simulink library "FMLibrary_v2"  (R2016b)
settings: Solver=ode45  StartTime=0.0  StopTime=10.0  RelTol=1e-3
undefined symbols (not defined in the file or in its folder): ActuatorStruct, drivePeakCurrent, IdxJoint, JointPositionGuardMax_rad, JointPositionGuardMin_rad, Lb, Lf, Lu, motorTorqueConstant, RobotStruct, sampleTime, transmissionRatio
undefined symbols (not defined in the file): JointAbsoluteEncoderCounts_rev
libraries: simulink x23, VariousBlocksLibrary x10, FM_Library x8, FMLibrary_v2 x5, simulink_extras x1
(part 2 of 2)

== system FMLibrary_v2/Utilities/Latch ==
  note: Enable == HIGH: OUtput follows input
      | Enable == LOW: Output does not change anymore.
  In : Inport
  Enable : EnablePort
  Out : Outport  InitialOutput=ic
  wires:
  In/1 -> Out/1

== system FMLibrary_v2/Utilities/LatchRising ==
  note: Enable == HIGH: OUtput follows input
      | Enable == LOW: Output does not change anymore.
  In : Inport
  Trigger : TriggerPort  VariantControl=Variant  PortDimensions=1
  Out : Outport  InitialOutput=ic
  wires:
  In/1 -> Out/1

== system FMLibrary_v2/Utilities/Stopwatch ==
  note: Stopwatch -
      | Outputs time in seconds.
      | Reset during high level of Rest pulse
  ResetHighActive : Inport
  Counter Free-Running : simulink/Sources/Counter Free-Running  NumBits=32  tsamp=-1
  Data Type Conversion : DataTypeConversion  OutDataTypeStr=double
  LatchRising : FM_Library/LatchRising  ic=0
  Subtract : Sum  Inputs=-+
  sample time : Gain  Gain=sampleTime
  Time_s : Outport
  wires:
  ResetHighActive/1 -> LatchRising/Trigger
  Data Type Conversion/1 -> sample time/1
  sample time/1 -> Time_s/1
  Subtract/1 -> Data Type Conversion/1
  Counter Free-Running/1 -> LatchRising/1, Subtract/2
  LatchRising/1 -> Subtract/1  "startTime"

== system FMLibrary_v2/Utilities/TorqueLimiter ==
  note: This block limits the Desird Torque to an interval [-TorqueLimit, +TorqueLimit]. It also sets TorqueGuardMax_Nm to 0.5 Nm more than the TorqueLimit. This is used in the DriveEnableLogic block to completely shut down the motor (and with that, all other motors) if the limit is severly (by 0.5 Nm) exceeded.
      |
      | Note that the actuators are rated to a maximum of 4 Nm, so if the user puts a TorqueLimit of higher than 4 Nm in, this block will still limit it to 4 Nm.
  Torque_Limit_Nm : Inport
  Torque_Des_Nm : Inport  Port=2
  AbsoluteMaximumTorque_Nm : Constant  Value=8
  Bias : Bias  Bias=0.5
  MinMax : MinMax  Inputs=2
  Saturation Dynamic : simulink/Discontinuities/Saturation Dynamic  OutMin=[]  OutMax=[]  OutDataTypeStr=Inherit: Same as second input  OutDataType=fixdt(1, 16)  OutScaling=2^-10  DoSatur=off
  Unary Minus : UnaryMinus
  Torque_GuardMax_Nm : Outport
  Torque_Des_Limited_Nm : Outport  Port=2
  wires:
  Torque_Limit_Nm/1 -> MinMax/1
  AbsoluteMaximumTorque_Nm/1 -> MinMax/2
  MinMax/1 -> Bias/1, Unary Minus/1, Saturation Dynamic/1
  Unary Minus/1 -> Saturation Dynamic/3
  Saturation Dynamic/1 -> Torque_Des_Limited_Nm/1
  Torque_Des_Nm/1 -> Saturation Dynamic/2
  Bias/1 -> Torque_GuardMax_Nm/1

== system FMLibrary_v2/DataFromEtherCAT_FM/Calculate//Arrange Joint and Op Space/forward kinematics ==
  JointPosition_rad : Inport  PortDimensions=[2 1]
  JointVelocity_rads : Inport  Port=2  PortDimensions=[2 1]
  JointAcceleration_rads2 : Inport  Port=3  PortDimensions=[2 1]
  Je : MATLAB Function  TreatAsAtomicUnit=on
  Jedot : MATLAB Function  TreatAsAtomicUnit=on
  Product : Product  Multiplication=Matrix(*)
  calculate xddot : MATLAB Function  TreatAsAtomicUnit=on
  forward kinematics : MATLAB Function  TreatAsAtomicUnit=on
  x : Outport
  xdot : Outport  Port=2
  xddot : Outport  Port=3
  J : Outport  Port=4
  Jdot : Outport  Port=5
  wires:
  JointPosition_rad/1 -> forward kinematics/1(q), Jedot/1(q), Je/1(q)
  Je/1(Je) -> calculate xddot/3(J), Product/1, J/1
  JointVelocity_rads/1 -> calculate xddot/2(qdot), Product/2, Jedot/2(qdot)
  Jedot/1(Jedot) -> calculate xddot/4(Jdot), Jdot/1
  Product/1 -> xdot/1
  forward kinematics/1(x) -> x/1
  calculate xddot/1(xddot) -> xddot/1
  JointAcceleration_rads2/1 -> calculate xddot/1(qddot)

== system FMLibrary_v2/DataToEtherCAT_FM/WorkspacePositionGuard/CreateSingleErrorValue ==
  ErrorChecks : Inport
  Data Type Conversion1 : DataTypeConversion  OutDataTypeStr=double
  Data Type Conversion2 : DataTypeConversion  OutDataTypeStr=int32
  MATLAB Function : MATLAB Function  TreatAsAtomicUnit=on
  error : Outport
  wires:
  MATLAB Function/1(out) -> Data Type Conversion2/1
  Data Type Conversion1/1 -> MATLAB Function/1(errors)
  ErrorChecks/1 -> Data Type Conversion1/1
  Data Type Conversion2/1 -> error/1

== system FMLibrary_v2/ToActuator/DriveEnableLogic/128_FromToActuatorConsistency ==
  note: This block checks whether the FromActuator and ToActuator blocks use the same ActuatorStruct. If not, you've done something wrong. It does this by checking if the JointEncoderOffsets are identical.
  To_ToActuator : Inport
  Bus Selector : BusSelector  OutputSignals=JointEncoderOffset
  Constant : Constant  Value=ActuatorStruct.JointEncoderOffset
  Relational Operator : RelationalOperator  Operator=~=  OutDataTypeStr=boolean  RndMeth=Nearest
  Error : Outport
  wires:
  To_ToActuator/1 -> Bus Selector/1
  Relational Operator/1 -> Error/1
  Bus Selector/1 -> Relational Operator/1  "<JointEncoderOffset>"
  Constant/1 -> Relational Operator/2

== system FMLibrary_v2/ToActuator/DriveEnableLogic/16_TorqueGuard ==
  To_ToActuator : Inport
  TorqueGuardMax : Inport  Port=2
  Abs : Abs
  Bus Selector : BusSelector  OutputSignals=JointTorque_Act_Nm
  Relational Operator : RelationalOperator  Operator=>  OutDataTypeStr=boolean  RndMeth=Nearest
  Error : Outport  PortDimensions=1
  wires:
  TorqueGuardMax/1 -> Relational Operator/2
  Bus Selector/1 -> Abs/1  "<JointTorque_Act_Nm>"
  To_ToActuator/1 -> Bus Selector/1
  Abs/1 -> Relational Operator/1
  Relational Operator/1 -> Error/1

== system FMLibrary_v2/ToActuator/DriveEnableLogic/1_ActuatorNotInUse ==
  note: When UseActuator = 0, this block outputs 1. Later in the chain, the ErrorValue is then negated, resulting in -1 if there are no other errors. Note, thus, that this output does not really indicate an error; more a status.
  UseActuator : Inport
  Logical Operator1 : Logic  Operator=NOT  AllPortsSameDT=off  OutDataTypeStr=boolean
  Error : Outport  PortDimensions=1
  wires:
  Logical Operator1/1 -> Error/1
  UseActuator/1 -> Logical Operator1/1

== system FMLibrary_v2/ToActuator/DriveEnableLogic/2_JointAnglePositionGuard ==
  note: This block makes sure that the motors are turned off (and cannot go on) when the joint is outside its normal range.
  To_ToActuator : Inport
  Bus Selector : BusSelector  OutputSignals=JointPosition_rad
  Logical Operator : Logic  Operator=OR  AllPortsSameDT=off  OutDataTypeStr=boolean
  Maximum : Constant  Value=JointPositionGuardMax_rad(IdxJoint)
  Minimum : Constant  Value=JointPositionGuardMin_rad(IdxJoint)
  Relational Operator : RelationalOperator  Operator=<=  OutDataTypeStr=boolean  RndMeth=Nearest
  Relational Operator1 : RelationalOperator  OutDataTypeStr=boolean  RndMeth=Nearest
  Error : Outport
  wires:
  To_ToActuator/1 -> Bus Selector/1
  Relational Operator/1 -> Logical Operator/1
  Relational Operator1/1 -> Logical Operator/2
  Logical Operator/1 -> Error/1
  Minimum/1 -> Relational Operator/2
  Maximum/1 -> Relational Operator1/2
  Bus Selector/1 -> Relational Operator1/1, Relational Operator/1  "<JointPosition_rad>"

== system FMLibrary_v2/ToActuator/DriveEnableLogic/32_EncoderConsistency ==
  note: This block checks whether the three encoders are consistent. Ideally, the sum (with jointAngle negated) should be exactly zero at all times (also when forces are exerted). We allow some room around it however.
  To_ToActuator : Inport
  Abs : Abs
  Add : Sum  Inputs=+-
  Bus Selector : BusSelector  OutputSignals=JointPosition_IncEnc_rad,JointPosition_AbsEnc_rad
  Compare To Constant : simulink/Logic and Bit Operations/Compare To Constant  relop=<=  const=3.0  OutDataTypeStr=boolean
  EncoderInConsistency_rad : Concatenate  NumInputs=1
  Error : Outport
  wires:
  Bus Selector/1 -> Add/1  "<JointPosition_IncEnc_rad>"
  To_ToActuator/1 -> Bus Selector/1
  Compare To Constant/1 -> Error/1
  Abs/1 -> Compare To Constant/1
  Bus Selector/2 -> Add/2  "<JointPosition_AbsEnc_rad>"
  Add/1 -> EncoderInConsistency_rad/1
  EncoderInConsistency_rad/1 -> Abs/1

== system FMLibrary_v2/ToActuator/DriveEnableLogic/64_DriveError ==
  note: This memory block is to avoid that this error 'turns on' when another error is triggered.
  note: This memory block is to avoid an
      | algebraic loop
  note: This block checks whether the drive went off by itself. Reasons why this could happen are: undervoltage of the motor power supply, short-circuit detection triggered, I2t error etc.
      | The first few seconds that the drive should be on (i.e., DriveEnable = True), the drive is in the process of turning on, and will not be really on. In order to avoid direct turn-off due to this, we disable this error the first few seconds.
  To_ToActuator : Inport
  DriveEnable : Inport  Port=2
  Bus Selector : BusSelector  OutputSignals=OperationEnabled
  CountHowLongEnableWasTrue : MATLAB Function  TreatAsAtomicUnit=on
  InhibitTime_s : Constant  Value=2.0
  Logical Operator : Logic  AllPortsSameDT=off  OutDataTypeStr=boolean
  Logical Operator2 : Logic  Operator=NOT  AllPortsSameDT=off  OutDataTypeStr=boolean
  Memory : Memory
  Memory1 : Memory
  Relational Operator : RelationalOperator  OutDataTypeStr=boolean  RndMeth=Nearest
  ToSeconds : Gain  Gain=sampleTime
  Error : Outport  PortDimensions=1
  wires:
  Logical Operator/1 -> Error/1
  To_ToActuator/1 -> Memory1/1
  Bus Selector/1 -> Logical Operator2/1  "<OperationEnabled>"
  DriveEnable/1 -> Memory/1
  CountHowLongEnableWasTrue/1(y) -> ToSeconds/1
  ToSeconds/1 -> Relational Operator/1
  Relational Operator/1 -> Logical Operator/1
  InhibitTime_s/1 -> Relational Operator/2
  Memory/1 -> CountHowLongEnableWasTrue/1(u)
  Memory1/1 -> Bus Selector/1
  Logical Operator2/1 -> Logical Operator/2

== system FMLibrary_v2/ToActuator/DriveEnableLogic/8_MotorAngleGuard ==
  note: This block checks whether the motor encoder gives sensible data, i.e., if the motor angle is within the expected range. The expected range is the full stroke of the output shaft plus the maximum spring deflection, transformed to motor angle space.
  To_ToActuator : Inport
  TorqueGuardMax : Inport  Port=2
  Add : Sum  Inputs=+-
  Add1 : Sum
  Bus Selector : BusSelector  OutputSignals=MotorPosition_IncEnc_rad
  Divide : Product  Inputs=*/
  Logical Operator : Logic  Operator=OR  AllPortsSameDT=off  OutDataTypeStr=boolean
  Maximum : Constant  Value=ActuatorStruct.JointAnglePositionGuardMax_rad
  Minimum : Constant  Value=ActuatorStruct.JointAnglePositionGuardMin_rad
  Relational Operator1 : RelationalOperator  Operator=<=  OutDataTypeStr=boolean  RndMeth=Nearest
  Relational Operator2 : RelationalOperator  OutDataTypeStr=boolean  RndMeth=Nearest
  SpringStiffness : Constant  Value=ActuatorStruct.SpringStiffness_Nm_rad
  TransformToMotorSpace : Gain  Gain=ActuatorStruct.gearboxRatio
  TransformToMotorSpace1 : Gain  Gain=ActuatorStruct.gearboxRatio
  Error : Outport
  wires:
  To_ToActuator/1 -> Bus Selector/1
  Bus Selector/1 -> Relational Operator2/1, Relational Operator1/1  "<MotorPosition_IncEnc_rad>"
  Relational Operator1/1 -> Logical Operator/1
  Relational Operator2/1 -> Logical Operator/2
  Logical Operator/1 -> Error/1
  TransformToMotorSpace1/1 -> Relational Operator1/2
  Add1/1 -> TransformToMotorSpace/1
  Add/1 -> TransformToMotorSpace1/1
  TransformToMotorSpace/1 -> Relational Operator2/2
  TorqueGuardMax/1 -> Divide/1
  SpringStiffness/1 -> Divide/2
  Maximum/1 -> Add1/1
  Divide/1 -> Add/2, Add1/2  "MaximumSpringDeflection_rad"
  Minimum/1 -> Add/1

== system FMLibrary_v2/ToActuator/DriveEnableLogic/CreateSingleErrorValue ==
  ErrorChecks : Inport
  Data Type Conversion1 : DataTypeConversion  OutDataTypeStr=double
  Data Type Conversion2 : DataTypeConversion  OutDataTypeStr=int32
  MATLAB Function : MATLAB Function  TreatAsAtomicUnit=on
  Select_NotUseActuator : Selector  InputPortWidth=3  IndexOptions=Index vector (dialog)  Indices=1  OutputSizes=1
  Switch : Switch  Criteria=u2 ~= 0
  Unary Minus : UnaryMinus
  Out1 : Outport
  wires:
  Data Type Conversion2/1 -> Switch/3, Unary Minus/1
  MATLAB Function/1(out) -> Data Type Conversion2/1
  Data Type Conversion1/1 -> MATLAB Function/1(errors), Select_NotUseActuator/1
  Select_NotUseActuator/1 -> Switch/2
  ErrorChecks/1 -> Data Type Conversion1/1
  Switch/1 -> Out1/1
  Unary Minus/1 -> Switch/1

== system FMLibrary_v2/ToActuator/DriveEnableLogic/LatchRising ==
  in : Inport
  Trigger : TriggerPort  VariantControl=Variant  PortDimensions=1
  out : Outport
  wires:
  in/1 -> out/1

== system FMLibrary_v2/ToActuator/DriveEnableLogic/LatchRising1 ==
  in : Inport
  Trigger : TriggerPort  VariantControl=Variant  PortDimensions=1
  out : Outport
  wires:
  in/1 -> out/1

== matlab function FMLibrary_v2/Utilities/FilterFourthOrder/Filter1 ==
  data: x input; OmegaFilter input; y output; sampleTime parameter
function y = Filter2ndOrder(x, OmegaFilter, sampleTime)
%#codegen

persistent yd_prev y_prev;
if isempty(yd_prev)
    yd_prev = 0; 
    y_prev = 0; %Derivative of the above signal
end;

% Do 2nd order filtering with given omega and zeta=0.7; input of filter
% is vel_inc_sampleTime_unfilt; output is y (we assign to vel_inc_s
% later). 
if OmegaFilter==0 || isinf(OmegaFilter)
    y=x;
    y_prev=y;
    yd_prev =0;
else
    zeta = 0.7;
    ydd = OmegaFilter^2 * (x - y_prev) - 2*zeta*OmegaFilter* yd_prev;
    yd = yd_prev + ydd * sampleTime;
    y = y_prev + yd * sampleTime;

    y_prev = y; yd_prev = yd;
end;

== matlab function FMLibrary_v2/FromActuator1/CalculateJointVelocity/FOAW ==
  data: x input; xdot output; sampleTime parameter; noise input
function xdot = foaw(x, sampleTime, noise)
%#codegen

SIZE = 100; % number of samples in buffer
NOISE = noise;
Ts = sampleTime;

persistent posbuffer;
persistent buffercntr;

% initialize buffer
if isempty(posbuffer)
    posbuffer = zeros(SIZE,1); % 1D case for now
    buffercntr = 0;
end

% fill buffer: shift data and add new value (loose oldest sample)
posbuffer = [posbuffer(2:end); x];
buffercntr = buffercntr + 1;
if buffercntr > SIZE, buffercntr = SIZE; end;

% if buffercntr = 1, only 1 data point is available, and you can't make a
% velocity prediction based on 1 data point. Set velocity ot 0, and return
% function
xdot = 0;
if buffercntr <= 3
    return;
end

for n = 1:buffercntr-1 % n = window size
        
    % step 2
    currentpos = posbuffer(end);

    % step 3 - calculate LS approximation of slope (hence velocity)
    b = n*sum(posbuffer(end-n:end)) - 2*sum(posbuffer(end-n:end).*(n:-1:0)');
    b = b / (Ts*n*(n+1)*(n+2)/6);

    % step 4 - check whether the line an + bn*Ts passes through all points inside the 
    % window within the uncertainty band of each point 
    jj = 0:n;
    yk_hat = currentpos-(b*jj*Ts);
    yk = posbuffer(end-jj)';
    if any(abs(yk_hat-yk) > NOISE)
        break;
    end

    xdot = b;
end

== matlab function FMLibrary_v2/DataToEtherCAT_FM/FTSensorError/MATLAB Function ==
  data: ForcesTorques input; e output; MaxForcesTorques input
function e = fcn(ForcesTorques, MaxForcesTorques)

% throw error when any of the forces/torques go over a max allowable value
if any(abs(ForcesTorques) > MaxForcesTorques) 
    e = 1;
else
    e = 0;
end

== matlab function FMLibrary_v2/Utilities/EncodeDesiredTorque ==
  data: MotorTorque_Des_IU output int16; JointTorque_Des_Nm input; transmissionRatio parameter; motorTorqueConstant parameter; drivePeakCurrent parameter
function MotorTorque_Des_IU = EncodeDesiredTorque(JointTorque_Des_Nm, transmissionRatio, motorTorqueConstant, drivePeakCurrent)
%#codegen
% Calculate the target torque in incremental units for a desired joint
% torque.

% compute torque at motor (negate because sign change due to transmission)
torque_motor = JointTorque_Des_Nm / transmissionRatio; 

% desired current (i_des) = torque_motor / kt (torque constant)
i_des = torque_motor / motorTorqueConstant;

% calculate the target torque in incremental units [IU], see CoE manual
% Technosoftmotion
MotorTorque_Des_IU = int16( 65520*i_des / (2*drivePeakCurrent) );

== matlab function FMLibrary_v2/Utilities/DecodeActualTorque ==
  data: JointTorque_Act_Nm output; MotorCurrent_Act_IU input int16; transmissionRatio parameter; drivePeakCurrent parameter; motorTorqueConstant parameter
function JointTorque_Act_Nm = DecodeActualTorque(MotorCurrent_Act_IU, transmissionRatio, drivePeakCurrent, motorTorqueConstant)
%#codegen
%

% convert incremental units to motor torque value. See the technosoft CoE
% manual for the decoding
torquemotor_act = motorTorqueConstant * (double(MotorCurrent_Act_IU)*2*drivePeakCurrent / 65520);

% motor torque to joint torque (transmission). Negate due to sign change
% due to transmission.
JointTorque_Act_Nm = torquemotor_act * transmissionRatio;

== matlab function FMLibrary_v2/Utilities/FilterFourthOrder/Filter2 ==
  data: x input; OmegaFilter input; y output; sampleTime parameter
function y = Filter2ndOrder(x, OmegaFilter, sampleTime)
%#codegen

persistent yd_prev y_prev;
if isempty(yd_prev)
    yd_prev = 0; 
    y_prev = 0; %Derivative of the above signal
end;

% Do 2nd order filtering with given omega and zeta=0.7; input of filter
% is vel_inc_sampleTime_unfilt; output is y (we assign to vel_inc_s
% later). 
if OmegaFilter==0 || isinf(OmegaFilter)
    y=x;
    y_prev=y;
    yd_prev =0;
else
    zeta = 0.7;
    ydd = OmegaFilter^2 * (x - y_prev) - 2*zeta*OmegaFilter* yd_prev;
    yd = yd_prev + ydd * sampleTime;
    y = y_prev + yd * sampleTime;

    y_prev = y; yd_prev = yd;
end;

== matlab function FMLibrary_v2/Controller/AFFC ==
  data: p output; t input; q input; qdot input; qddot input; e input; tau output; Lf parameter; Lu parameter; Lb parameter; w input
function [p,tau] = fcn(t, q, qdot, qddot, e, Lf, Lu, Lb,w)

persistent p_;

if isempty(p_)
%     p_ = [0.00173;0.00159;0.048;0.07889;-0.00389;0.08784;-0.00474];
    p_ = zeros(7,1);
end


% inverse kinematics & jacobians
% q = func_eq_IK(x(1),x(2),Lf,Lu,Lb);
J = func_eq_Je(q(1),q(2),Lf,Lu,Lb);
% qdot = pinv(J)*xdot;
Jdot = func_eq_Jedot(q(1),q(2),qdot(1),qdot(2),Lf,Lu,Lb);
% qddot = pinv(J)*(xddot-Jdot*qdot);

% create Psi
Psi = [diag([qddot(1) qddot(2)]) J'*J*qddot+J'*Jdot*qdot [sign(qdot(1)) qdot(1); 0 0] [0 0;sign(qdot(2)) qdot(2)] ];

% learning matrix Gamma
eta = 0.95*exp(-t/150) + 0.05;
% eta = 1;
% wI = 1e-3;
% wme = 5e-2;
% wfd = 1e-3;
% wfs = 1e-3;

wI = w(1);
wme = w(2);
wfd = w(3);
wfs = w(4);

Gamma = eta*diag([wI wI wme wfs wfd wfs wfd]);

% update p (parameter vector)

% learning rule
dp = Gamma*Psi'*e;

p_ = p_ + dp;

% Psi = [diag([qddot(1) qddot(2)]) J'*J*qddot+J'*Jdot*qdot [ssign(qdot(1)) qdot(1); 0 0] [0 0;ssign(qdot(2)) qdot(2)] ];


% feedforward torque
tau = Psi*p_;

p = p_;

function y = ssign(u,beta)

if nargin == 1
    beta = 150;
end

y = 2./(1+exp(-beta*u))-1;

== stateflow chart FMLibrary_v2/StateMachineLocal/SystemLocalStateMachine ==
  settings: initializeOutput=1
  state Operational
    state Calibration
      en:
      systemState = 2;
      velBelowThreshold = false;
      du:
      velBelowThreshold = checkVelThreshold(0.001 );
      state JointVelLarge
      state JointVelSmall
      state DoCalibration
        en: systemState = 201;
      state CalibrationDone
        en: systemState = 299;
      (default) -> JointVelLarge
      JointVelSmall -> JointVelLarge [order 1] : [!velBelowThreshold]
      JointVelLarge -> JointVelSmall : [velBelowThreshold]
      JointVelSmall -> DoCalibration [order 2] : after(2,sec)
      DoCalibration -> CalibrationDone
    state Homing
      en:
      systemState = reqSystemState;
      isAtHome = false;
      du:
      isAtHome = checkEndpointPosition(homeLocationSize);
      state NotAtHome
      state AtHome
      state HomingDone
        en: systemState = 399;
      (default) -> NotAtHome
      AtHome -> NotAtHome [order 1] : [!isAtHome]
      NotAtHome -> AtHome : [isAtHome]
      AtHome -> HomingDone [order 2] : after(1,sec)
    state Run
      en: systemState = 4;
    (default) -> Calibration
    CalibrationDone -> Homing : [reqSystemState == 301 || reqSystemState == 302]
    Run -> Homing : [reqSystemState==3]
    HomingDone -> Run : [reqSystemState==4]
  state Idle
    en:
    systemState = 0;
  state Init
    en:
    systemState = 1;
    du:
    isInitialized = true;
  state Error
    en: systemState=-1;
  (default) -> Idle
  Init -> Operational [order 1] : [isInitialized]
  Idle -> Init [order 2] : [reqSystemState==1]
  Init -> Idle [order 3] : [reqSystemState==0]
  Error -> Idle : [!error   && reqSystemState==0]
  Init -> Error [order 2] : [error]
  Idle -> Error [order 1] : [error]
  Operational -> Idle [order 2] : [reqSystemState==0]
  Operational -> Error [order 1] : [error]
  data: threshold function_input double; velIsUnderThreshold function_output boolean; threshold function_input double; isAtEndpoint function_output boolean; reqSystemState input double; currentSystemState output double; error input boolean; x input double; xdot input double; HomePosition input double; isAtHome local boolean; velBelowThreshold local boolean; isInitialized local double; homeLocationSize input
  function velIsUnderThreshold = checkVelThreshold(threshold):
    | function velIsUnderThreshold = checkVelThreshold(threshold)
    |  
    | velIsUnderThreshold = all(abs(xdot) <= threshold);
  function isAtEndpoint = checkEndpointPosition(threshold):
    | function isAtEndpoint = checkEndpointPosition(threshold)
    | % check whether the endpoint position is within a specified circle with
    | % radius threshold and midopoint HomePosition
    | 
    | % calculate distance between home position and joint positions
    | d = sqrt(sum((HomePosition - x).^2));
    | 
    | if imag(d) || isinf(d) || isnan(d)
    |     isAtEndpoint = false;
    | else
    |     isAtEndpoint = d <= threshold;
    | end

== matlab function FMLibrary_v2/StateMachineLocal/MATLAB Function ==
  data: stateChanged input; state input; systemStateChanged output
function systemStateChanged  = fcn(stateChanged,state)

systemStateChanged = 0;


if stateChanged
    switch(state)
        case 201 % do calibration
            systemStateChanged = 1;
    end
end

== matlab function FMLibrary_v2/Utilities/EndstopAndSafety/MATLAB Function ==
  data: deltaX input; v_limit output; MaxAcc input; ReturnVelocity input; ReturnVelocitySlope input
function v_limit = fcn(deltaX, MaxAcc, ReturnVelocity,ReturnVelocitySlope)
% Note: all input parameters should be positive!
% deltaX should be positive while in the 'allowed' region. If needed,
% negate the input to get it such.
%
% For the output: the v_limit is positive when in the 'allowed' region. if
% needed, negate the output to get it such.

%#codegen

if deltaX>=0
    v_limit = sqrt(2*MaxAcc * deltaX);
else
    v_limit = max ([deltaX*ReturnVelocitySlope, -ReturnVelocity]); 
end;

== matlab function FMLibrary_v2/Utilities/EndstopAndSafety/MATLAB Function1 ==
  data: deltaX input; v_limit output; MaxAcc input; ReturnVelocity input; ReturnVelocitySlope input
function v_limit = fcn(deltaX, MaxAcc, ReturnVelocity,ReturnVelocitySlope)
% Note: all input parameters should be positive!
% deltaX should be positive while in the 'allowed' region. If needed,
% negate the input to get it such.
%
% For the output: the v_limit is positive when in the 'allowed' region. if
% needed, negate the output to get it such.

%#codegen

if deltaX>=0
    v_limit = sqrt(2*MaxAcc * deltaX);
else
    v_limit = max ([deltaX*ReturnVelocitySlope, -ReturnVelocity]); 
end;

== matlab function FMLibrary_v2/ToActuator/DriveEnableLogic/64_DriveError/CountHowLongEnableWasTrue ==
  data: u input; y output
function y = fcn(u)
%#codegen
%
% This block counts how many samples the input has been on (true). As soon
% as the input goes false, the counter is reset.
persistent onCounter;

if isempty(onCounter)
    onCounter = 0;
end;

if u == 1
    onCounter = onCounter + 1;
else
    % u == 0
    onCounter = 0;
end;
y = onCounter;

== matlab function FMLibrary_v2/FromActuator1/CalibrateMotorPosition     ==
  data: JointPosition_IncEnc_rad output; MotorPosition_rad input; MotorPositionCalibrated_rad output; transmissionRatio parameter; JointPosition_AbsEnc_rad input; Calibrate input
function [JointPosition_IncEnc_rad,MotorPositionCalibrated_rad]...
    = CalibrateMotorPosition( MotorPosition_rad, transmissionRatio, JointPosition_AbsEnc_rad, Calibrate)
%#codegen

% This block includes calibration such that (ideally) the motor angle is
% zero when the joint angle and spring deflection are zero as well. Before
% the calibration has occurred, the output of this function is -1e9*. This
% is chosen such that the value is always outside the allowed motor angle
% range; this prevents the drive from being allowed to turn on.
% 
% * I wanted to use -inf as starting function, but I'm not sure whether
%   that will be handled correctly in all cases.

persistent isCalibrated;
persistent offset;

if isempty(isCalibrated) % no calibration needed
    isCalibrated = 1;
    offset = 0;
end;


if Calibrate
%     if ~isempty(JointPosition_AbsEnc_rad)
        target_pos_mot_rad = transmissionRatio * JointPosition_AbsEnc_rad; % This is what we should read
%         target_pos_mot_rad = CalibrationAngle; % This is what we should read / fix for now
        offset = target_pos_mot_rad - MotorPosition_rad; % calculate offset
%     else
%         % no absolute encoder data available, offset is zero
%         offset = 0;
%     end
    isCalibrated = 1;
end;

% if already calibrated, calculate calibrated motor angle
if isCalibrated
    MotorPositionCalibrated_rad = MotorPosition_rad + offset;
    JointPosition_IncEnc_rad = MotorPositionCalibrated_rad / transmissionRatio;
else
    MotorPositionCalibrated_rad = MotorPosition_rad;
    JointPosition_IncEnc_rad = MotorPositionCalibrated_rad / transmissionRatio;
end;

== matlab function FMLibrary_v2/ToActuator/DriveEnableLogic/CreateSingleErrorValue/MATLAB Function ==
  data: errors input; out output
function out = errorToPowerOf2(errors)
%#codegen

% if size(errors,1) > size(errors,2)
%     errors = errors.';
% end
out = sum(errors.*(2.^(0:(length(errors)-1)).'));

== matlab function FMLibrary_v2/DataFromEtherCAT_FM/Calculate//Arrange Joint and Op Space/forward kinematics/Je ==
  data: q input; Je output size=[2 2]; Lf parameter; Lu parameter; Lb parameter
function Je = Je( q, Lf, Lu, Lb)
%#codegen

% Calculate the Jacobian for this particular device configuration.
% Note that the function func_eq_Je needs to be in the libraries/kinematis_functions folder

% jacobians
Je = func_eq_Je(q(1),q(2),Lf,Lu,Lb);

== matlab function FMLibrary_v2/DataFromEtherCAT_FM/Calculate//Arrange Joint and Op Space/forward kinematics/Jedot ==
  data: q input; qdot input; Jedot output size=[2 2]; Lf parameter; Lu parameter; Lb parameter
function Jedot = Jedot( q, qdot, Lf, Lu, Lb)
%#codegen

% Calculate the time derivative of the Jacobian for this particular device configuration.
% Note that the function func_eq_Je needs to be in the libraries/kinematis_functions folder


% jacobians
Jedot = func_eq_Jedot(q(1),q(2),qdot(1),qdot(2),Lf,Lu,Lb);

== matlab function FMLibrary_v2/DataFromEtherCAT_FM/FTSensor_K6D27/CorrectOffset ==
  data: u_in input; u_out output; reset input; corrected output
function [u_out,corrected] = CorrectOffset(u_in,reset)
%#codegen

persistent data_ offset_ counter_ corrected_;
N = 1000;

% initialize
if isempty(data_)
    data_ = zeros(size(u_in,1), N);
    offset_ = zeros(size(u_in));
    counter_ = 1;
    corrected_ = 0;
end

if (counter_ <= N)
    data_(:,counter_) = u_in;
end

counter_ = counter_ + 1;
if reset
    counter_ = 1;
end

% calculate mean
if counter_ == N
    corrected_ = 1;
    offset_ = mean(data_,2);
end

corrected = corrected_;
u_out = u_in - offset_;

== matlab function FMLibrary_v2/FromActuator1/CheckOperationEnabled ==
  data: u input; y output
function y = fcn(u)
%#codegen

mask  = bin2dec('0000000001101111');
match = bin2dec('0000000000100111');

masked = bitand(u,mask);
if masked==match
    y=1;
else
    y=0;
end;

== matlab function FMLibrary_v2/DataFromEtherCAT_FM/Calculate//Arrange Joint and Op Space/IK all joints ==
  data: x input; q_all output; Lf parameter; Lu parameter; Lb parameter
function q_all = IK_all(x,Lf,Lu,Lb)
%#codegen

if (x(2) >= 0.07)
    q_all = func_eqs_IK_all(x(1),x(2),Lf,Lu,Lb);
else
    x = [0;0.07];
    q_all = func_eqs_IK_all(x(1),x(2),Lf,Lu,Lb);
end

== matlab function FMLibrary_v2/DataFromEtherCAT_FM/Calculate//Arrange Joint and Op Space/forward kinematics/calculate xddot ==
  data: qddot input; qdot input size=[2 1]; J input; xddot output size=[2 1]; Jdot input
function xddot = calc_xddot(qddot, qdot, J, Jdot)
%#codegen

xddot = J*qddot + Jdot*qdot;

== matlab function FMLibrary_v2/DataFromEtherCAT_FM/Calculate//Arrange Joint and Op Space/forward kinematics/forward kinematics ==
  data: q input; x output size=[2 1]; Lf parameter; Lu parameter; Lb parameter
function x = FK(q, Lf, Lu, Lb)
%#codegen

% Calculate the endpoint position (forward kinematics)
% Note that the function func_eq_FK needs to be in the libraries/kinematis_functions folder


x = func_eq_FK(q(1),q(2),Lf,Lu,Lb);

== matlab function FMLibrary_v2/ToActuator/DriveEnableLogic/enableDrive (CoE) ==
  data: ControlWord output; enable input; TimePerState_ms input
function ControlWord = enabledrive(enable, TimePerState_ms)
%#codegen
%
% Input arguments:
% enable:
%   0: Disable drive
%   Any non-zero: enable drive.
% TimePerState_ms:
%   A four-element array containing the time in ms for each state (states
%   are: 0, 128, 6, 7. The final state, 15, is kept until drive needs to be
%   disabled again.
%
% Changing enable forces the initialize-sequence to run
persistent previousEnable;
persistent counter;
if isempty(previousEnable)
    previousEnable = enable; % No enabling of the drive at startup
    counter = 1e6;
end;

if enable~=previousEnable
    counter = 0;
end;
previousEnable = enable;

TimePerState_cum = cumsum(TimePerState_ms);

if enable~=0
    counter = counter+1;
    if counter < TimePerState_cum(1);
        ControlWord_ = 0;
    elseif counter < TimePerState_cum(2);
        ControlWord_ = 128;
    elseif counter < TimePerState_cum(3);
        ControlWord_ = 6;
    elseif counter < TimePerState_cum(4);
        ControlWord_ = 7;
    else
        ControlWord_ = 15;
    end
else
    ControlWord_ = 6;
end

ControlWord = uint16(ControlWord_);

== matlab function FMLibrary_v2/ToActuator/EncodeDesiredTorque ==
  data: MotorTorque_Des_IU output int16; JointTorque_Des_Nm input; transmissionRatio parameter; motorTorqueConstant parameter; drivePeakCurrent parameter
function MotorTorque_Des_IU = EncodeDesiredTorque(JointTorque_Des_Nm, transmissionRatio, motorTorqueConstant, drivePeakCurrent)
%#codegen
% Calculate the target torque in incremental units for a desired joint
% torque.

% compute torque at motor (negate because sign change due to transmission)
torque_motor = JointTorque_Des_Nm / transmissionRatio; 

% desired current (i_des) = torque_motor / kt (torque constant)
i_des = torque_motor / motorTorqueConstant;

% calculate the target torque in incremental units [IU], see CoE manual
% Technosoftmotion
MotorTorque_Des_IU = int16( 65520*i_des / (2*drivePeakCurrent) );

== matlab function FMLibrary_v2/FromActuator1/DecodeActualTorque ==
  data: JointTorque_Act_Nm output; MotorCurrent_Act_IU input int16; transmissionRatio parameter; drivePeakCurrent parameter; motorTorqueConstant parameter
function JointTorque_Act_Nm = DecodeActualTorque(MotorCurrent_Act_IU, transmissionRatio, drivePeakCurrent, motorTorqueConstant)
%#codegen
%

% convert incremental units to motor torque value. See the technosoft CoE
% manual for the decoding
torquemotor_act = motorTorqueConstant * (double(MotorCurrent_Act_IU)*2*drivePeakCurrent / 65520);

% motor torque to joint torque (transmission). Negate due to sign change
% due to transmission.
JointTorque_Act_Nm = torquemotor_act * transmissionRatio;

== matlab function FMLibrary_v2/FromActuator1/DecodeEncoder_AbsEnc ==
  data: Encoder_counts input; EncoderCounts_rev parameter; EncoderPosition_rad output
function EncoderPosition_rad = ...
    DecodeEncoder(Encoder_counts, EncoderCounts_rev)
%#codegen

% This block decodes the motor encoder counts to the motor angle

EncoderPosition_rad = (double(Encoder_counts) / EncoderCounts_rev * 2 * pi);

== matlab function FMLibrary_v2/FromActuator1/DecodeEncoder_IncEnc ==
  data: Encoder_counts input; EncoderCounts_rev parameter; EncoderPosition_rad output
function EncoderPosition_rad = ...
    DecodeEncoder(Encoder_counts, EncoderCounts_rev)
%#codegen

% This block decodes the motor encoder counts to the motor angle

EncoderPosition_rad = (double(Encoder_counts) / EncoderCounts_rev * 2 * pi);

== matlab function FMLibrary_v2/FromActuator1/CalibrateAbsEncoder ==
  data: encoderPosition input; JointPosition_AbsEnc_rad output; offset input
function JointPosition_AbsEnc_rad = CalibrateAbsoluteEncoder(encoderPosition, offset)
%#codegen

% unwrap encoder angle (in case the encoder goes through 0
encoderPosition = unwrap(encoderPosition);

% remove offset
JointPosition_AbsEnc_rad = encoderPosition - offset;

% since the absolute encoder is mounted upside-down, negate the
% jointposition angle
JointPosition_AbsEnc_rad = -JointPosition_AbsEnc_rad;

== matlab function FMLibrary_v2/Controller/run/IK ==
  data: q output; x input; xdot input; xddot input; qdot output; Lf parameter; Lu parameter; Lb parameter; qddot output
function [q,qdot,qddot] = fcn(x,xdot,xddot, Lf, Lu, Lb)


% inverse kinematics & jacobians
q = func_eq_IK(x(1),x(2),Lf,Lu,Lb);
J = func_eq_Je(q(1),q(2),Lf,Lu,Lb);
qdot = pinv(J)*xdot;
Jdot = func_eq_Jedot(q(1),q(2),qdot(1),qdot(2),Lf,Lu,Lb);
qddot = pinv(J)*(xddot-Jdot*qdot);

== matlab function FMLibrary_v2/Controller/run/reference ==
  data: t input; p output; v output; a output; T input; n input; hstart input; hend input; wstart input; wend input
function [p,v,a] = fcn(t,T,n,hstart,hend,wstart,wend)
%#codegen

% T = 80;
% hstart = 0.02;
% hend = 0.02;
% n = 5;
% wstart = 0.5;%0.2*2*pi;
% wend = 0.5;%0.2*2*pi;

p = func_p_hypothrochoid(t,T,n,hstart,hend,wstart,wend);
v = func_v_hypothrochoid(t,T,n,hstart,hend,wstart,wend);
a = func_a_hypothrochoid(t,T,n,hstart,hend,wstart,wend);

== matlab function FMLibrary_v2/DataFromEtherCAT_FM/FTSensor_K6D27/SensorOutputToForce1 ==
  data: FT output; u input; calibrationMatrix input; offset input
function FT = VtoF(u, calibrationMatrix, offset)
%#codegen

% ME supplies a zero offset voltages. If 
if ~isempty(offset)
    u = u + offset;
end

% Calculate forces and torques (in sensor space)
FT = calibrationMatrix*u;

== matlab function FMLibrary_v2/DataFromEtherCAT_FM/FTSensor_K6D27/SensorToOperationalSpace ==
  data: q_all input; Fs input; FTOpSpace output
function FTOpSpace = ForceSensorToOperationalSpace(q_all,Fs)
%#codegen

% select correct angles. Note! During assembly we weren't very consistent
% to which forearm the sensor is fixed. For FM1 (green), the sensor is
% attached to arm 2, hence the rotation matrics are made using angles
% theta1 and theta2
% rotation matrices (I derived them from actuator 1 to endpoint, but
% transformation is other way around (i.e. inverse). Since inverse calculation 
% could take some time, Could be done by
% negating the angles instead of inverse of matrix.
theta1 = theta_all(1);
theta2 = (pi-theta_all(2)); % pi-theta2 since theta2 is the internal angle of this joint

R = [-cos(theta1+theta2) sin(theta1+theta2);-sin(theta1+theta2) -cos(theta1+theta2)];

% transform force
FTOpSpace = R*Fs(1:2);

== matlab function FMLibrary_v2/DataToEtherCAT_FM/WorkspacePositionGuard/CheckForSingularity ==
  data: J input; kappa output
function kappa = conditionnumber(J)
%#codegen

kappa = norm(pinv(J))*norm(J);

== matlab function FMLibrary_v2/DataToEtherCAT_FM/WorkspacePositionGuard/CheckInternalAngles ==
  data: theta input; angleError output; isCalibrated input
function angleError = checkInternalErrors(theta,isCalibrated)
%#codegen

angleError = 0;

if isCalibrated
    % check whether theta2 or theta4 are smaller than 0.95*pi. If larger, throw
    % error
    if any(theta([2 4]) >= 0.95*pi)
        angleError = 1;
    end
end

== matlab function FMLibrary_v2/DataToEtherCAT_FM/WorkspacePositionGuard/CreateSingleErrorValue/MATLAB Function ==
  data: errors input; out output
function out = errorToPowerOf2(errors)
%#codegen

% if size(errors,1) > size(errors,2)
%     errors = errors.';
% end
out = sum(errors.*(2.^(0:(length(errors)-1)).'));

== matlab function FMLibrary_v2/DataToEtherCAT_FM/WorkspacePositionGuard/EndpointPositionGuard ==
  data: xe input; error output; correctState input
function error = fcn(xe, correctState)
%#codegen


error = 0;

% only check workspace boundaries after homing state is done
if ~correctState 
    return; 
end

% x0 = 0;
% y0 = 0.2354;
% a = 0.11;
% b = 0.08;

% workspace (see design document)
x0 = 0;
y0 = 0.25024;
a = 0.1746;
b = 0.13;%0.1048;

% check if endpoint is outside a predefined ellipse
x = xe(1);
y = xe(2);

% workspace is defined as an ellipse
e = (x-x0)^2 / a^2 + (y-y0)^2 / b^2;

% if is larger than 1, the endpoint is outside the workspace
if e > 1
    error = 1;
end

== matlab function FMLibrary_v2/Utilities/FOAW ==
  data: x input; xdot output; sampleTime parameter; noise input
function xdot = foaw(x, sampleTime, noise)
%#codegen

SIZE = 100; % number of samples in buffer
NOISE = noise;
Ts = sampleTime;

persistent posbuffer;
persistent buffercntr;

% initialize buffer
if isempty(posbuffer)
    posbuffer = zeros(SIZE,1); % 1D case for now
    buffercntr = 0;
end

% fill buffer: shift data and add new value (loose oldest sample)
posbuffer = [posbuffer(2:end); x];
buffercntr = buffercntr + 1;
if buffercntr > SIZE, buffercntr = SIZE; end;

% if buffercntr = 1, only 1 data point is available, and you can't make a
% velocity prediction based on 1 data point. Set velocity ot 0, and return
% function
xdot = 0;
if buffercntr <= 3
    return;
end

for n = 1:buffercntr-1 % n = window size
        
    % step 2
    currentpos = posbuffer(end);

    % step 3 - calculate LS approximation of slope (hence velocity)
    b = n*sum(posbuffer(end-n:end)) - 2*sum(posbuffer(end-n:end).*(n:-1:0)');
    b = b / (Ts*n*(n+1)*(n+2)/6);

    % step 4 - check whether the line an + bn*Ts passes through all points inside the 
    % window within the uncertainty band of each point 
    jj = 0:n;
    yk_hat = currentpos-(b*jj*Ts);
    yk = posbuffer(end-jj)';
    if any(abs(yk_hat-yk) > NOISE)
        break;
    end

    xdot = b;
end

== matlab function FMLibrary_v2/Utilities/DecodeEncoder ==
  data: Encoder_counts input; EncoderCounts_rev parameter; EncoderPosition_rad output
function EncoderPosition_rad = ...
    DecodeEncoder(Encoder_counts, EncoderCounts_rev)
%#codegen

% This block decodes the motor encoder counts to the motor angle

EncoderPosition_rad = (double(Encoder_counts) / EncoderCounts_rev * 2 * pi);
